simulink library "Velocity"  (Simulink 8.2)
settings: Solver=ode45  StartTime=0.0  StopTime=10.0  RelTol=1e-3
libraries: carnot x1
settings Model: Creator=lena.frank  LastModifiedBy=drhf

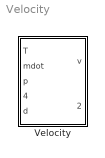
== system Velocity ==
  Velocity : Subsystem  mask(velocity){}
      mask help: Calculates the velocity in a pipe [m/s] assuming a round pipe. The diameter is taken from the THV-vector.
      mask Help: web(fullfile(path_carnot('help'),'Velocity.html'),'-helpbrowser')

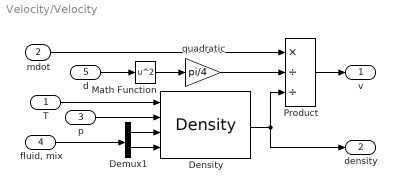
== system Velocity/Velocity ==
  T : Inport
  mdot : Inport  Port=2
  p : Inport  Port=3
  "fluid, mix" : Inport  Port=4
  d : Inport  Port=5
  Demux1 : Demux  Outputs=2
  Density : carnot/Basic/Material_Properties/Density  VariantControl=CarlibClassic  INPUTARGUMENTS=state variables (classic)  DEBUGLEVEL=DEBUGLEVEL  MAXTOTALWARNINGS=inf  MAXCONSECUTIVEWARNINGS=inf  WRITETOFILE=0  FILENAME='errors.txt'
  Math Function : Math  Operator=square  SaturateOnIntegerOverflow=on
  Product : Product  Inputs=*//  SaturateOnIntegerOverflow=on  InputSameDT=on  OutDataTypeStr=Inherit: Same as first input
  quadratic : Gain  Gain=pi/4  SaturateOnIntegerOverflow=on  OutDataTypeStr=Inherit: Same as input  ParamDataTypeStr=Inherit: Same as input
  v : Outport
  density : Outport  Port=2
  wires:
  Density/1 -> density/1, Product/3
  quadratic/1 -> Product/2
  Math Function/1 -> quadratic/1
  d/1 -> Math Function/1
  Product/1 -> v/1
  T/1 -> Density/1
  Demux1/2 -> Density/4
  mdot/1 -> Product/1
  Demux1/1 -> Density/3
  "fluid, mix"/1 -> Demux1/1
  p/1 -> Density/2
